simulink model "threeDiskOscillatorRig"  (R2021a)
settings: Solver=VariableStepAuto  StartTime=0.0  StopTime=simTime  RelTol=1e-8
values from neighbouring files (symbols this model uses):
  atan_scale = 100    [MandatoryAssignmentB_Loopsyn.m]    (also in MandatoryAssignmentB_Q13.m; MandatoryAssignmentB_Q9.m; threeDiskOscillator_9.m)
  b_1 = mean(ECP_values([6 7]))    [MandatoryAssignmentB_Loopsyn.m]    (also in MandatoryAssignmentB_Q13.m; MandatoryAssignmentB_Q9.m; threeDiskOscillator_9.m)
  b_2 = mean(ECP_values([8 9]))    [MandatoryAssignmentB_Loopsyn.m]    (also in MandatoryAssignmentB_Q13.m; MandatoryAssignmentB_Q9.m; threeDiskOscillator_9.m)
  b_3 = mean(ECP_values([10 11]))    [MandatoryAssignmentB_Loopsyn.m]    (also in MandatoryAssignmentB_Q13.m; MandatoryAssignmentB_Q9.m; threeDiskOscillator_9.m)
  B_change = [1 0;0 0]    [threeDiskOscillator_9.m]
  C = double(jacobian(g, x))    [MandatoryAssignmentB_Loopsyn.m]    (also in MandatoryAssignmentB_Q13.m; MandatoryAssignmentB_Q9.m; threeDiskOscillator_9.m)
  C_aug = [C zeros(3, 1)]    [threeDiskOscillator_9.m]
  detect_time = f_u_time + 3.75    (= 28.75)    [threeDiskOscillator_9.m]
  F_aug = [F_d E ... (first row only)    [threeDiskOscillator_9.m]
  f_m = [0;-0.025;0]    [threeDiskOscillator_9.m]
  f_m_time = 8.5    [threeDiskOscillator_9.m]
  f_u = [0;0]    [threeDiskOscillator_9.m]
  f_u_time = 25    [threeDiskOscillator_9.m]
  G_aug = [G_d; zeros(1, 2)]    [threeDiskOscillator_9.m]
  h = chi2inv(1 - P_F, 1)/2    [threeDiskOscillator_9.m]
  J_1 = 0.0325    [MandatoryAssignmentB_Loopsyn.m]    (also in MandatoryAssignmentB_Q13.m; MandatoryAssignmentB_Q15.m = ECP_values(1); MandatoryAssignmentB_Q9.m = ECP_values(1); threeDiskOscillator_9.m = ECP_values(1))
  J_2 = ECP_values(2)    [MandatoryAssignmentB_Loopsyn.m]    (also in MandatoryAssignmentB_Q13.m; MandatoryAssignmentB_Q9.m; threeDiskOscillator_9.m)
  J_3 = ECP_values(3)    [MandatoryAssignmentB_Loopsyn.m]    (also in MandatoryAssignmentB_Q13.m; MandatoryAssignmentB_Q9.m; threeDiskOscillator_9.m)
  k_1 = ECP_values(4)    [MandatoryAssignmentB_Loopsyn.m]    (also in MandatoryAssignmentB_Q13.m; MandatoryAssignmentB_Q9.m; threeDiskOscillator_9.m)
  k_2 = ECP_values(5)    [MandatoryAssignmentB_Loopsyn.m]    (also in MandatoryAssignmentB_Q13.m; MandatoryAssignmentB_Q9.m; threeDiskOscillator_9.m)
  L_aug = dlqe(F_aug,eye(7),C_aug,1e-3*eye(7),deg2rad(0.0056)*eye(3))    [threeDiskOscillator_9.m]
  sigma_meas = 0.0093*eye(3)    [threeDiskOscillator_9.m]
  T_Cm = ECP_values(13)    [MandatoryAssignmentB_Loopsyn.m]    (also in MandatoryAssignmentB_Q13.m; MandatoryAssignmentB_Q9.m; threeDiskOscillator_9.m)
  T_Cp = ECP_values(12)    [MandatoryAssignmentB_Loopsyn.m]    (also in MandatoryAssignmentB_Q13.m; MandatoryAssignmentB_Q9.m; threeDiskOscillator_9.m)
  T_s = 0.004    [MandatoryAssignmentB_Q13.m]    (also in MandatoryAssignmentB_Q14.m = 0.0004; MandatoryAssignmentB_Q14_RP.m = 0.0004; MandatoryAssignmentB_Q14_messy.m = 0.0004; MandatoryAssignmentB_Q9.m)
  u_fault = 0    [threeDiskOscillator_9.m]
  w_th = 0.75    [MandatoryAssignmentB_Loopsyn.m]    (also in MandatoryAssignmentB_Q13.m; MandatoryAssignmentB_Q9.m; threeDiskOscillator_9.m)
  x_0 = [0;0;0;0;0;0]    [MandatoryAssignmentB_Q14.m]    (also in MandatoryAssignmentB_Q14_RP.m; MandatoryAssignmentB_Q14_messy.m; MandatoryAssignmentB_Q9.m; threeDiskOscillator_9.m)
libraries: simulink x1
settings Model: Creator=dimpa  LastModifiedBy=dimpa
settings SolverCC: AlgebraicLoopSolver=TrustRegion
settings DataIOCC: ReturnWorkspaceOutputs=off
settings DebuggingCC: SFMachineParentedDataDiag=warning  ArithmeticOperatorsInVariantConditions=warning
settings SFSimCC: SimUseLocalCustomCode=off  CustomCodeUndefinedFunction=UseInterfaceOnly
settings RTWCC: RTWUseLocalCustomCode=off

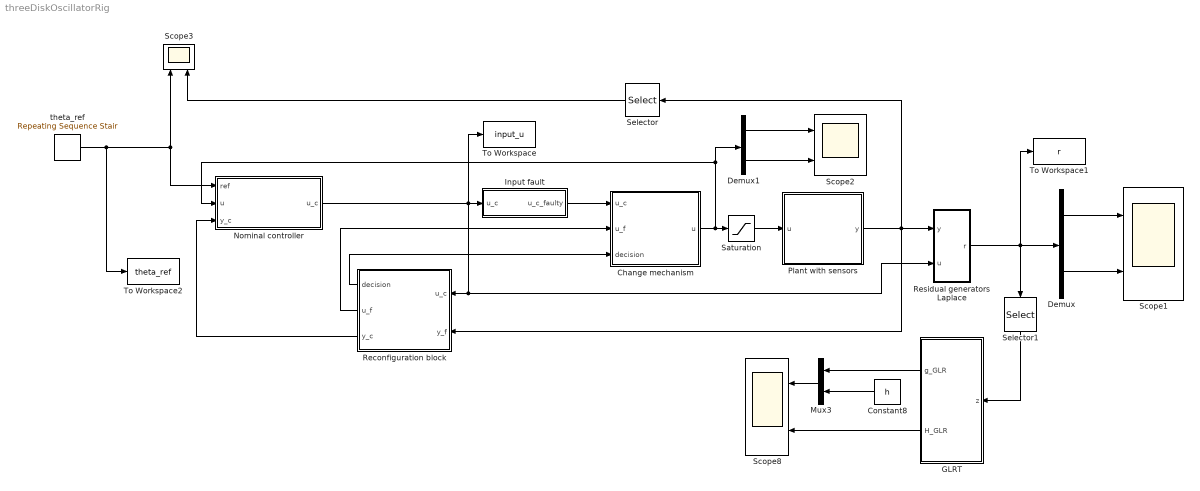
== system threeDiskOscillatorRig ==
  Change mechanism : Subsystem
  Constant8 : Constant  Value=h
  Demux : Demux  Outputs=2
  Demux1 : Demux  Outputs=2
  GLRT : Subsystem
  Input fault : Subsystem
  Mux3 : Mux  Inputs=2
  Nominal controller : Subsystem
  Plant with sensors : Subsystem
  Reconfiguration block : Subsystem
  Residual generators Laplace : Subsystem
  Saturation : Saturate  UpperLimit=2  LowerLimit=-2
  Scope{1..3,8} (4 alike) : Scope  NumInputPorts=2
  Selector : Selector  InputPortWidth=3  IndexOptions=Index vector (dialog)  Indices=[3]  OutputSizes=1
  Selector1 : Selector  InputPortWidth=2  IndexOptions=Index vector (dialog)  Indices=[2]  OutputSizes=1
  To Workspace : ToWorkspace  VariableName=input_u  SaveFormat=Timeseries  SampleTime=T_s
  To Workspace1 : ToWorkspace  VariableName=r  SaveFormat=Timeseries  SampleTime=T_s
  To Workspace2 : ToWorkspace  VariableName=theta_ref  SaveFormat=Timeseries  SampleTime=T_s
  theta_ref : simulink/Sources/Repeating Sequence Stair  OutValues=[0 1.57 0]  tsamp=5  OutMin=[]  OutMax=[]  OutDataTypeStr=double  OutputDataTypeScalingMode=double  OutDataType=fixdt(0,8)  ConRadixGroup=Best Precision: Vector-wise  OutScaling=2^-12
  wires:
  Selector/1 -> Scope3/2
  Saturation/1 -> Plant with sensors/1(u)
  theta_ref/1 -> Nominal controller/1(ref), Scope3/1, To Workspace2/1
  Plant with sensors/1(y) -> Reconfiguration block/2(y_f), Residual generators Laplace/1(y), Selector/1
  Residual generators Laplace/1(r) -> Selector1/1, Demux/1, To Workspace1/1
  GLRT/1(g_GLR) -> Mux3/1
  GLRT/2(H_GLR) -> Scope8/2
  Constant8/1 -> Mux3/2
  Mux3/1 -> Scope8/1
  Selector1/1 -> GLRT/1(z)
  Demux/1 -> Scope1/1
  Demux/2 -> Scope1/2
  Demux1/1 -> Scope2/1
  Demux1/2 -> Scope2/2
  Nominal controller/1(u_c) -> Input fault/1(u_c), Residual generators Laplace/2(u), Reconfiguration block/1(u_c), To Workspace/1
  Reconfiguration block/3(y_c) -> Nominal controller/3(y_c)
  Change mechanism/1(u) -> Nominal controller/2(u), Demux1/1, Saturation/1
  Input fault/1(u_c_faulty) -> Change mechanism/1(u_c)
  Reconfiguration block/1(decision) -> Change mechanism/3(decision)
  Reconfiguration block/2(u_f) -> Change mechanism/2(u_f)

== system threeDiskOscillatorRig/Change mechanism ==
  u_c : Inport
  u_f : Inport  Port=2
  decision : Inport  Port=3
  Gain2 : Gain  Gain=B_change  Multiplication=Matrix(K*u) (u vector)
  Switch2 : Switch  OutDataTypeStr=double
  u : Outport
  wires:
  Gain2/1 -> Switch2/3
  decision/1 -> Switch2/2
  u_c/1 -> Switch2/1
  Switch2/1 -> u/1
  u_f/1 -> Gain2/1

== system threeDiskOscillatorRig/GLRT ==
  z : Inport
  g_GLR : Outport  VectorParamsAs1DForOutWhenUnconnected=off
  H_GLR : Outport  Port=2  VectorParamsAs1DForOutWhenUnconnected=off

== system threeDiskOscillatorRig/Input fault ==
  u_c : Inport
  Sum4 : Sum  Inputs=|++
  f_u : Step  Time=f_u_time  After=f_u  SampleTime=0
  u_c_faulty : Outport
  wires:
  f_u/1 -> Sum4/2
  u_c/1 -> Sum4/1
  Sum4/1 -> u_c_faulty/1

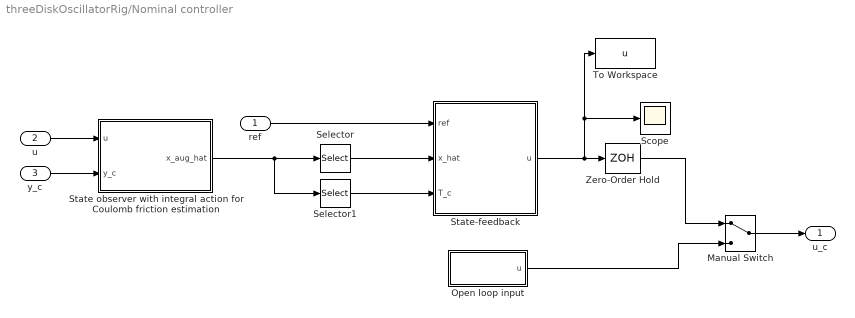
== system threeDiskOscillatorRig/Nominal controller ==
  ref : Inport
  u : Inport  Port=2
  y_c : Inport  Port=3
  Manual Switch : ManualSwitch
  Open loop input : Subsystem
  Scope : Scope
  Selector : Selector  InputPortWidth=7  IndexOptions=Index vector (dialog)  Indices=[1:6]  OutputSizes=1
  Selector1 : Selector  InputPortWidth=7  IndexOptions=Index vector (dialog)  Indices=[7]  OutputSizes=1
  State observer with integral action for Coulomb friction estimation : Subsystem
  State-feedback : Subsystem
  To Workspace : ToWorkspace  VariableName=u  SaveFormat=Timeseries  SampleTime=T_s
  Zero-Order Hold : ZeroOrderHold  SampleTime=T_s
  u_c : Outport
  wires:
  Zero-Order Hold/1 -> Manual Switch/1
  y_c/1 -> State observer with integral action for Coulomb friction estimation/2(y_c)
  u/1 -> State observer with integral action for Coulomb friction estimation/1(u)
  Open loop input/1(u) -> Manual Switch/2
  Manual Switch/1 -> u_c/1
  Selector/1 -> State-feedback/2(x_hat)
  Selector1/1 -> State-feedback/3(T_c)
  State observer with integral action for Coulomb friction estimation/1(x_aug_hat) -> Selector1/1, Selector/1
  ref/1 -> State-feedback/1(ref)
  State-feedback/1(u) -> To Workspace/1, Scope/1, Zero-Order Hold/1

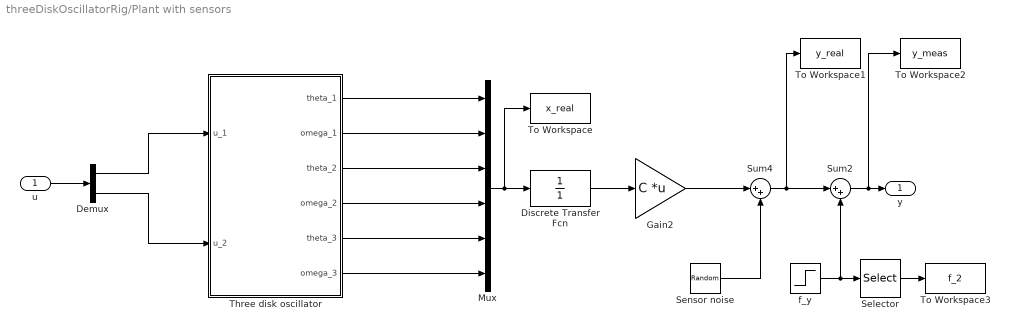
== system threeDiskOscillatorRig/Plant with sensors ==
  u : Inport
  Demux : Demux  Outputs=2
  Discrete Transfer Fcn : DiscreteTransferFcn  Denominator=[1]  SampleTime=T_s
  Gain2 : Gain  Gain=C  Multiplication=Matrix(K*u) (u vector)
  Mux : Mux  Inputs=6
  Selector : Selector  InputPortWidth=3  IndexOptions=Index vector (dialog)  Indices=[2]  OutputSizes=1
  Sensor noise : RandomNumber  Mean=zeros(3,1)  Variance=diag(sigma_meas^2)  SampleTime=T_s
  Sum2 : Sum  Inputs=|++
  Sum4 : Sum  Inputs=|++
  Three disk oscillator : Subsystem
  To Workspace : ToWorkspace  VariableName=x_real  SaveFormat=Timeseries  SampleTime=T_s
  To Workspace1 : ToWorkspace  VariableName=y_real  SaveFormat=Timeseries  SampleTime=T_s
  To Workspace2 : ToWorkspace  VariableName=y_meas  SaveFormat=Timeseries  SampleTime=T_s
  To Workspace3 : ToWorkspace  VariableName=f_2  SaveFormat=Timeseries  SampleTime=T_s
  f_y : Step  Time=f_m_time  Before=[0;0;0]  After=f_m  SampleTime=0
  y : Outport  VectorParamsAs1DForOutWhenUnconnected=off
  wires:
  u/1 -> Demux/1
  Three disk oscillator/2(omega_1) -> Mux/2
  Three disk oscillator/1(theta_1) -> Mux/1
  Mux/1 -> To Workspace/1, Discrete Transfer Fcn/1
  Three disk oscillator/4(omega_2) -> Mux/4
  Three disk oscillator/3(theta_2) -> Mux/3
  Discrete Transfer Fcn/1 -> Gain2/1
  Gain2/1 -> Sum4/1
  Sum4/1 -> To Workspace1/1, Sum2/1
  Sensor noise/1 -> Sum4/2
  Three disk oscillator/6(omega_3) -> Mux/6
  Three disk oscillator/5(theta_3) -> Mux/5
  f_y/1 -> Sum2/2, Selector/1
  Sum2/1 -> To Workspace2/1, y/1
  Selector/1 -> To Workspace3/1
  Demux/1 -> Three disk oscillator/1(u_1)
  Demux/2 -> Three disk oscillator/2(u_2)

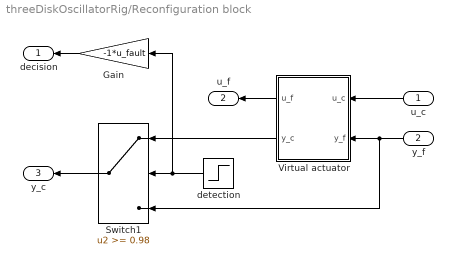
== system threeDiskOscillatorRig/Reconfiguration block ==
  u_c : Inport
  y_f : Inport  Port=2
  Gain : Gain  Gain=-1*u_fault
  Switch1 : Switch  Threshold=0.98
  Virtual actuator : Subsystem
  detection : Step  Time=detect_time  SampleTime=T_s
  decision : Outport  VectorParamsAs1DForOutWhenUnconnected=off
  u_f : Outport  Port=2  VectorParamsAs1DForOutWhenUnconnected=off
  y_c : Outport  Port=3  VectorParamsAs1DForOutWhenUnconnected=off
  wires:
  u_c/1 -> Virtual actuator/1(u_c)
  detection/1 -> Gain/1, Switch1/2
  Switch1/1 -> y_c/1
  Virtual actuator/2(y_c) -> Switch1/1
  y_f/1 -> Virtual actuator/2(y_f), Switch1/3
  Virtual actuator/1(u_f) -> u_f/1
  Gain/1 -> decision/1

== system threeDiskOscillatorRig/Residual generators Laplace ==
  y : Inport
  u : Inport  Port=2
  Demux : Demux  Outputs=3
  Demux1 : Demux  Outputs=2
  Mux : Mux  Inputs=2
  r : Outport  VectorParamsAs1DForOutWhenUnconnected=off
  wires:
  y/1 -> Demux/1
  Mux/1 -> r/1
  u/1 -> Demux1/1

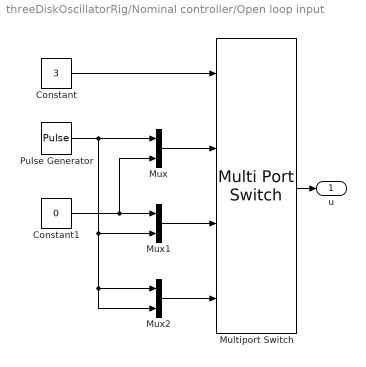
== system threeDiskOscillatorRig/Nominal controller/Open loop input ==
  Constant : Constant  Value=3
  Constant1 : Constant  Value=0
  Multiport Switch : MultiPortSwitch
  Mux : Mux  Inputs=2
  Mux1 : Mux  Inputs=2
  Mux2 : Mux  Inputs=2
  Pulse Generator : DiscretePulseGenerator  PulseType=Time based  Period=10  PulseWidth=5
  u : Outport
  wires:
  Constant1/1 -> Mux1/1, Mux/2
  Pulse Generator/1 -> Mux2/2, Mux2/1, Mux1/2, Mux/1
  Constant/1 -> Multiport Switch/1
  Mux2/1 -> Multiport Switch/4
  Mux/1 -> Multiport Switch/2
  Multiport Switch/1 -> u/1
  Mux1/1 -> Multiport Switch/3

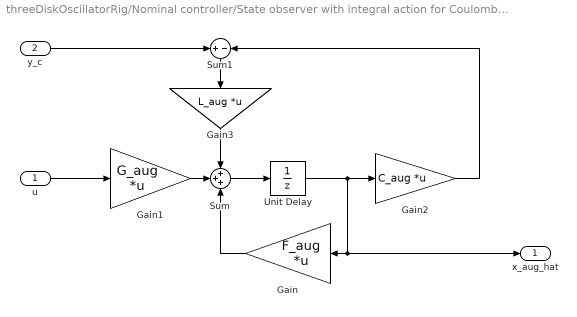
== system threeDiskOscillatorRig/Nominal controller/State observer with integral action for Coulomb friction estimation ==
  u : Inport
  y_c : Inport  Port=2
  Gain : Gain  Gain=F_aug  Multiplication=Matrix(K*u) (u vector)
  Gain1 : Gain  Gain=G_aug  Multiplication=Matrix(K*u) (u vector)
  Gain2 : Gain  Gain=C_aug  Multiplication=Matrix(K*u) (u vector)
  Gain3 : Gain  Gain=L_aug  Multiplication=Matrix(K*u) (u vector)
  Sum : Sum  Inputs=+++
  Sum1 : Sum  Inputs=+-
  Unit Delay : UnitDelay  SampleTime=T_s  HasFrameUpgradeWarning=on
  x_aug_hat : Outport  VectorParamsAs1DForOutWhenUnconnected=off
  wires:
  Unit Delay/1 -> x_aug_hat/1, Gain/1, Gain2/1
  y_c/1 -> Sum1/1
  Sum1/1 -> Gain3/1
  Sum/1 -> Unit Delay/1
  Gain2/1 -> Sum1/2
  u/1 -> Gain1/1
  Gain1/1 -> Sum/2
  Gain/1 -> Sum/3
  Gain3/1 -> Sum/1

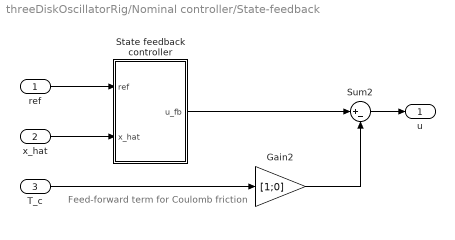
== system threeDiskOscillatorRig/Nominal controller/State-feedback ==
  note: Feed-forward term for Coulomb friction
  ref : Inport
  x_hat : Inport  Port=2
  T_c : Inport  Port=3
  Gain2 : Gain  Gain=[1;0]
  State feedback controller : Subsystem
  Sum2 : Sum  Inputs=|+-
  u : Outport  VectorParamsAs1DForOutWhenUnconnected=off
  wires:
  T_c/1 -> Gain2/1
  Gain2/1 -> Sum2/2
  Sum2/1 -> u/1
  ref/1 -> State feedback controller/1(ref)
  x_hat/1 -> State feedback controller/2(x_hat)
  State feedback controller/1(u_fb) -> Sum2/1

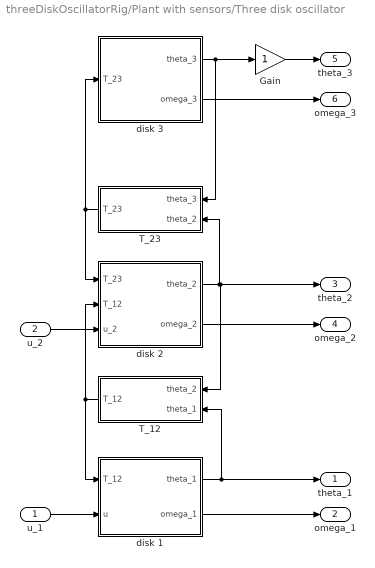
== system threeDiskOscillatorRig/Plant with sensors/Three disk oscillator ==
  u_1 : Inport
  u_2 : Inport  Port=2
  Gain : Gain
  T_12 : Subsystem
  T_23 : Subsystem
  disk 1 : Subsystem
  disk 2 : Subsystem
  disk 3 : Subsystem
  theta_1 : Outport  VectorParamsAs1DForOutWhenUnconnected=off
  omega_1 : Outport  Port=2  VectorParamsAs1DForOutWhenUnconnected=off
  theta_2 : Outport  Port=3  VectorParamsAs1DForOutWhenUnconnected=off
  omega_2 : Outport  Port=4  VectorParamsAs1DForOutWhenUnconnected=off
  theta_3 : Outport  Port=5  VectorParamsAs1DForOutWhenUnconnected=off
  omega_3 : Outport  Port=6  VectorParamsAs1DForOutWhenUnconnected=off
  wires:
  T_23/1(T_23) -> disk 2/1(T_23), disk 3/1(T_23)
  disk 1/1(theta_1) -> T_12/2(theta_1), theta_1/1
  disk 2/1(theta_2) -> T_23/2(theta_2), theta_2/1, T_12/1(theta_2)
  T_12/1(T_12) -> disk 1/1(T_12), disk 2/2(T_12)
  disk 3/2(omega_3) -> omega_3/1
  disk 1/2(omega_1) -> omega_1/1
  disk 2/2(omega_2) -> omega_2/1
  u_1/1 -> disk 1/2(u)
  disk 3/1(theta_3) -> Gain/1, T_23/1(theta_3)
  Gain/1 -> theta_3/1
  u_2/1 -> disk 2/3(u_2)

== system threeDiskOscillatorRig/Reconfiguration block/Virtual actuator ==
  u_c : Inport
  y_f : Inport  Port=2
  u_f : Outport  VectorParamsAs1DForOutWhenUnconnected=off
  y_c : Outport  Port=2  VectorParamsAs1DForOutWhenUnconnected=off

== system threeDiskOscillatorRig/Nominal controller/State-feedback/State feedback controller ==
  ref : Inport
  x_hat : Inport  Port=2
  u_fb : Outport

== system threeDiskOscillatorRig/Plant with sensors/Three disk oscillator/T_12 ==
  theta_2 : Inport
  theta_1 : Inport  Port=2
  Gain : Gain  Gain=k_1
  Sum : Sum  Inputs=|+-
  T_12 : Outport  VectorParamsAs1DForOutWhenUnconnected=off
  wires:
  theta_2/1 -> Sum/2
  theta_1/1 -> Sum/1
  Sum/1 -> Gain/1
  Gain/1 -> T_12/1

== system threeDiskOscillatorRig/Plant with sensors/Three disk oscillator/T_23 ==
  theta_3 : Inport
  theta_2 : Inport  Port=2
  Gain : Gain  Gain=k_2
  Sum : Sum  Inputs=-+|
  T_23 : Outport  VectorParamsAs1DForOutWhenUnconnected=off
  wires:
  Gain/1 -> T_23/1
  Sum/1 -> Gain/1
  theta_3/1 -> Sum/1
  theta_2/1 -> Sum/2

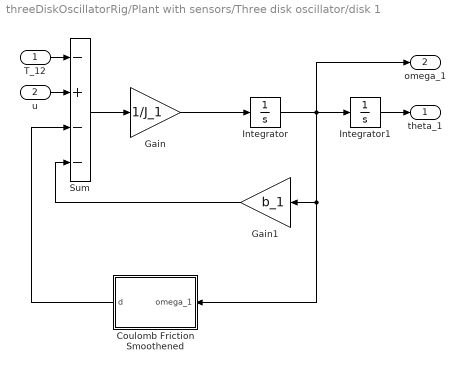
== system threeDiskOscillatorRig/Plant with sensors/Three disk oscillator/disk 1 ==
  T_12 : Inport
  u : Inport  Port=2
  Coulomb Friction Smoothened : Subsystem
  Gain : Gain  Gain=1/J_1
  Gain1 : Gain  Gain=b_1
  Integrator : Integrator  InitialCondition=x_0(2)
  Integrator1 : Integrator  InitialCondition=x_0(1)
  Sum : Sum  Inputs=-+--
  theta_1 : Outport  VectorParamsAs1DForOutWhenUnconnected=off
  omega_1 : Outport  Port=2  VectorParamsAs1DForOutWhenUnconnected=off
  wires:
  Sum/1 -> Gain/1
  Integrator/1 -> Integrator1/1, omega_1/1, Coulomb Friction Smoothened/1(omega_1), Gain1/1
  Gain1/1 -> Sum/4
  Integrator1/1 -> theta_1/1
  T_12/1 -> Sum/1
  u/1 -> Sum/2
  Gain/1 -> Integrator/1
  Coulomb Friction Smoothened/1(d) -> Sum/3

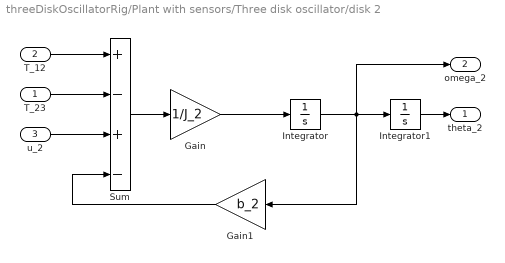
== system threeDiskOscillatorRig/Plant with sensors/Three disk oscillator/disk 2 ==
  T_23 : Inport
  T_12 : Inport  Port=2
  u_2 : Inport  Port=3
  Gain : Gain  Gain=1/J_2
  Gain1 : Gain  Gain=b_2
  Integrator : Integrator  InitialCondition=x_0(4)
  Integrator1 : Integrator  InitialCondition=x_0(3)
  Sum : Sum  Inputs=+-+-
  theta_2 : Outport  VectorParamsAs1DForOutWhenUnconnected=off
  omega_2 : Outport  Port=2  VectorParamsAs1DForOutWhenUnconnected=off
  wires:
  T_23/1 -> Sum/2
  T_12/1 -> Sum/1
  Integrator1/1 -> theta_2/1
  Gain1/1 -> Sum/4
  Gain/1 -> Integrator/1
  Integrator/1 -> Integrator1/1, Gain1/1, omega_2/1
  Sum/1 -> Gain/1
  u_2/1 -> Sum/3

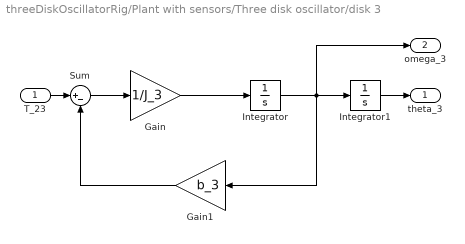
== system threeDiskOscillatorRig/Plant with sensors/Three disk oscillator/disk 3 ==
  T_23 : Inport
  Gain : Gain  Gain=1/J_3
  Gain1 : Gain  Gain=b_3
  Integrator : Integrator  InitialCondition=x_0(6)
  Integrator1 : Integrator  InitialCondition=x_0(5)
  Sum : Sum  Inputs=|+-
  theta_3 : Outport  VectorParamsAs1DForOutWhenUnconnected=off
  omega_3 : Outport  Port=2  VectorParamsAs1DForOutWhenUnconnected=off
  wires:
  Sum/1 -> Gain/1
  Integrator/1 -> Integrator1/1, omega_3/1, Gain1/1
  Gain/1 -> Integrator/1
  Gain1/1 -> Sum/2
  Integrator1/1 -> theta_3/1
  T_23/1 -> Sum/1

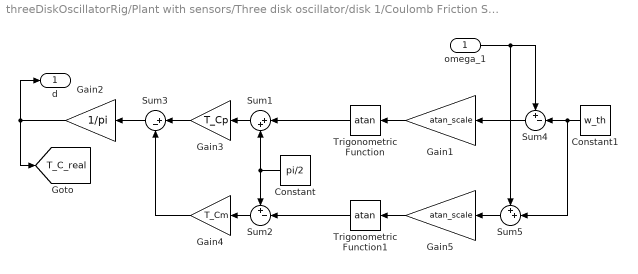
== system threeDiskOscillatorRig/Plant with sensors/Three disk oscillator/disk 1/Coulomb Friction Smoothened ==
  omega_1 : Inport
  Constant : Constant  Value=pi/2
  Constant1 : Constant  Value=w_th
  Gain1 : Gain  Gain=atan_scale
  Gain2 : Gain  Gain=1/pi
  Gain3 : Gain  Gain=T_Cp
  Gain4 : Gain  Gain=T_Cm
  Gain5 : Gain  Gain=atan_scale
  Sum1 : Sum  Inputs=|++
  Sum2 : Sum  Inputs=+-|
  Sum3 : Sum  Inputs=|+-
  Sum4 : Sum  Inputs=+-|
  Sum5 : Sum  Inputs=++|
  Trigonometric Function : Trigonometry  Operator=atan
  Trigonometric Function1 : Trigonometry  Operator=atan
  d : Outport  VectorParamsAs1DForOutWhenUnconnected=off
  tag scope: T_C_real=global
  wires:
  Gain1/1 -> Trigonometric Function/1
  Sum1/1 -> Gain3/1
  Constant/1 -> Sum2/1, Sum1/2
  Sum2/1 -> Gain4/1
  Sum3/1 -> Gain2/1
  Trigonometric Function/1 -> Sum1/1
  Gain4/1 -> Sum3/2
  Gain2/1 -> [T_C_real], d/1
  omega_1/1 -> Sum5/1, Sum4/1
  Gain3/1 -> Sum3/1
  Sum4/1 -> Gain1/1
  Constant1/1 -> Sum5/2, Sum4/2
  Gain5/1 -> Trigonometric Function1/1
  Sum5/1 -> Gain5/1
  Trigonometric Function1/1 -> Sum2/2
